simulink model "objselect"  (R2016a)
settings: Solver=VariableStepAuto  StartTime=0.0  StopTime=10.0  RelTol=1e-3
settings Model: Creator=NBGD  LastModifiedBy=NBGD

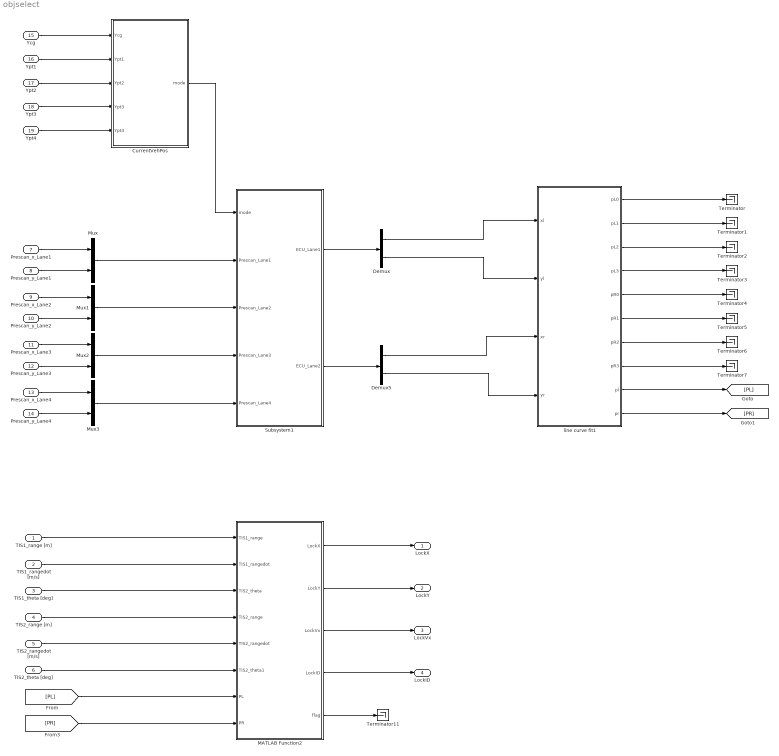
== system objselect ==
  TIS1_range [m] : Inport
  TIS1_rangedot [m/s] : Inport  Port=2
  TIS1_theta [deg] : Inport  Port=3
  TIS2_range [m] : Inport  Port=4
  TIS2_rangedot [m/s] : Inport  Port=5
  TIS2_theta [deg] : Inport  Port=6
  Prescan_x_Lane1 : Inport  Port=7
  Prescan_y_Lane1 : Inport  Port=8
  Prescan_x_Lane2 : Inport  Port=9
  Prescan_y_Lane2 : Inport  Port=10
  Prescan_x_Lane3 : Inport  Port=11
  Prescan_y_Lane3 : Inport  Port=12
  Prescan_x_Lane4 : Inport  Port=13
  Prescan_y_Lane4 : Inport  Port=14
  Ycg : Inport  Port=15
  Ypt1 : Inport  Port=16
  Ypt2 : Inport  Port=17
  Ypt3 : Inport  Port=18
  Ypt4 : Inport  Port=19
  CurrentVehPos : Subsystem
  Demux : Demux  Outputs=2
  Demux5 : Demux  Outputs=2
  MATLAB Function2 : MATLAB Function  TreatAsAtomicUnit=on
  Mux{,1..3} (4 alike) : Mux  Inputs=2
  Subsystem1 : Subsystem
  Terminator{,1..7,11} (9 alike) : Terminator
  line curve fit1 : MATLAB Function  TreatAsAtomicUnit=on
  LockX : Outport
  LockY : Outport  Port=2
  LockVx : Outport  Port=3
  LockID : Outport  Port=4
  wires:
  CurrentVehPos/1(mode) -> Subsystem1/1(mode)
  Demux/2 -> line curve fit1/2(yl)
  Demux5/2 -> line curve fit1/4(yr)
  Demux/1 -> line curve fit1/1(xl)
  Subsystem1/2(ECU_Lane2) -> Demux5/1
  line curve fit1/1(pL0) -> Terminator/1
  line curve fit1/2(pL1) -> Terminator1/1
  line curve fit1/3(pL2) -> Terminator2/1
  line curve fit1/4(pL3) -> Terminator3/1
  line curve fit1/5(pR0) -> Terminator4/1
  line curve fit1/6(pR1) -> Terminator5/1
  line curve fit1/7(pR2) -> Terminator6/1
  line curve fit1/8(pR3) -> Terminator7/1
  line curve fit1/9(pl) -> [PL]
  line curve fit1/10(pr) -> [PR]
  TIS1_range [m]/1 -> MATLAB Function2/1(TIS1_range)
  TIS1_rangedot [m/s]/1 -> MATLAB Function2/2(TIS1_rangedot)
  TIS1_theta [deg]/1 -> MATLAB Function2/3(TIS2_theta)
  TIS2_range [m]/1 -> MATLAB Function2/4(TIS2_range)
  TIS2_rangedot [m/s]/1 -> MATLAB Function2/5(TIS2_rangedot)
  TIS2_theta [deg]/1 -> MATLAB Function2/6(TIS2_theta1)
  MATLAB Function2/5(flag) -> Terminator11/1
  Prescan_x_Lane1/1 -> Mux/1
  Prescan_y_Lane1/1 -> Mux/2
  Mux/1 -> Subsystem1/2(Prescan_Lane1)
  Prescan_x_Lane2/1 -> Mux1/1
  Prescan_y_Lane2/1 -> Mux1/2
  Mux1/1 -> Subsystem1/3(Prescan_Lane2)
  Prescan_x_Lane3/1 -> Mux2/1
  Prescan_y_Lane3/1 -> Mux2/2
  Prescan_x_Lane4/1 -> Mux3/1
  Prescan_y_Lane4/1 -> Mux3/2
  Mux2/1 -> Subsystem1/4(Prescan_Lane3)
  Mux3/1 -> Subsystem1/5(Prescan_Lane4)
  Subsystem1/1(ECU_Lane1) -> Demux/1
  Demux5/1 -> line curve fit1/3(xr)
  [PL] -> MATLAB Function2/7(PL)
  [PR] -> MATLAB Function2/8(PR)
  MATLAB Function2/1(LockX) -> LockX/1
  MATLAB Function2/2(LockY) -> LockY/1
  MATLAB Function2/4(LockID) -> LockID/1
  MATLAB Function2/3(LockVx) -> LockVx/1
  Ycg/1 -> CurrentVehPos/1(Ycg)
  Ypt1/1 -> CurrentVehPos/2(Ypt1)
  Ypt2/1 -> CurrentVehPos/3(Ypt2)
  Ypt3/1 -> CurrentVehPos/4(Ypt3)
  Ypt4/1 -> CurrentVehPos/5(Ypt4)

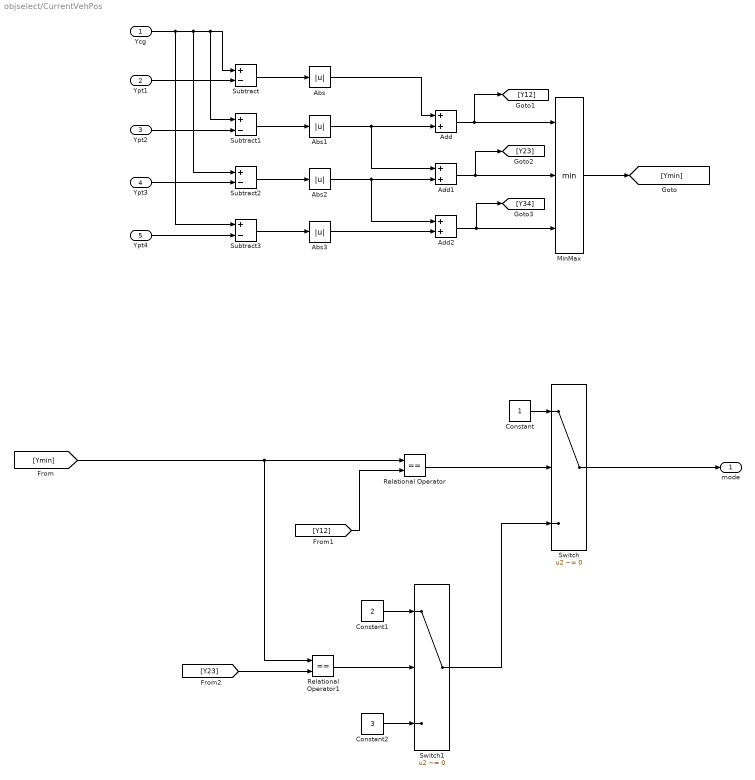
== system objselect/CurrentVehPos ==
  Ycg : Inport
  Ypt1 : Inport  Port=2
  Ypt2 : Inport  Port=3
  Ypt3 : Inport  Port=4
  Ypt4 : Inport  Port=5
  Abs{,1..3} (4 alike) : Abs
  Add : Sum
  Add1 : Sum
  Add2 : Sum
  Constant : Constant
  Constant1 : Constant  Value=2
  Constant2 : Constant  Value=3
  MinMax : MinMax  Inputs=3
  Relational Operator : RelationalOperator  Operator===  OutDataTypeStr=boolean
  Relational Operator1 : RelationalOperator  Operator===  OutDataTypeStr=boolean
  Subtract{,1..3} (4 alike) : Sum  Inputs=+-
  Switch : Switch  Criteria=u2 ~= 0
  Switch1 : Switch  Criteria=u2 ~= 0
  mode : Outport
  wires:
  Ycg/1 -> Subtract3/1, Subtract2/1, Subtract1/1, Subtract/1
  Abs/1 -> Add/1
  Ypt1/1 -> Subtract/2
  Subtract/1 -> Abs/1
  Ypt2/1 -> Subtract1/2
  Ypt3/1 -> Subtract2/2
  Ypt4/1 -> Subtract3/2
  Subtract2/1 -> Abs2/1
  Subtract3/1 -> Abs3/1
  Subtract1/1 -> Abs1/1
  Abs1/1 -> Add1/1, Add/2
  Abs2/1 -> Add2/1, Add1/2
  Abs3/1 -> Add2/2
  Add1/1 -> [Y23], MinMax/2
  Add/1 -> [Y12], MinMax/1
  Add2/1 -> [Y34], MinMax/3
  MinMax/1 -> [Ymin]
  Constant/1 -> Switch/1
  [Ymin] -> Relational Operator1/1, Relational Operator/1
  [Y12] -> Relational Operator/2
  Relational Operator/1 -> Switch/2
  Switch1/1 -> Switch/3
  Constant1/1 -> Switch1/1
  Relational Operator1/1 -> Switch1/2
  [Y23] -> Relational Operator1/2
  Constant2/1 -> Switch1/3
  Switch/1 -> mode/1

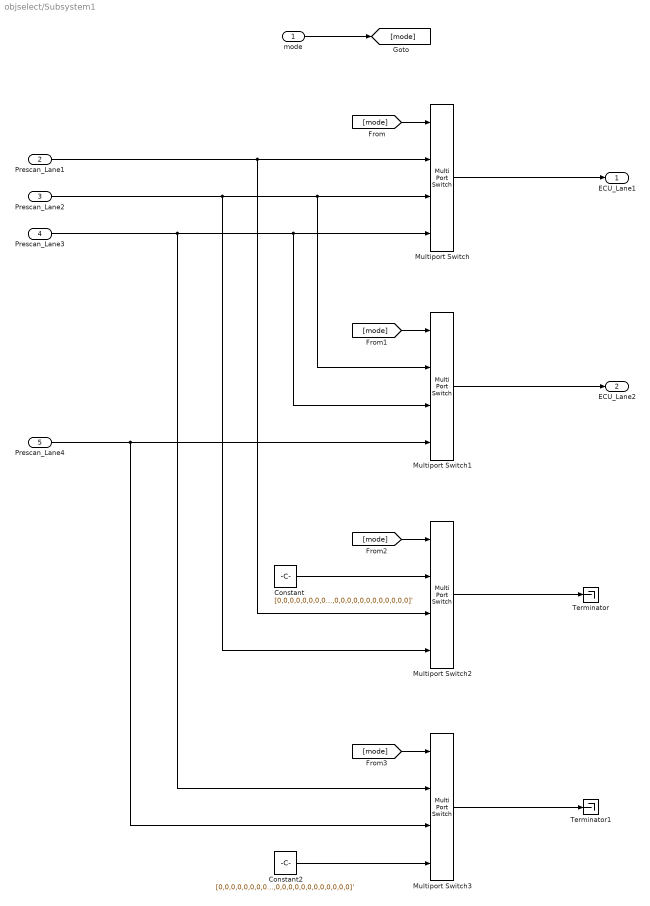
== system objselect/Subsystem1 ==
  mode : Inport
  Prescan_Lane1 : Inport  Port=2
  Prescan_Lane2 : Inport  Port=3
  Prescan_Lane3 : Inport  Port=4
  Prescan_Lane4 : Inport  Port=5
  Constant : Constant  Value=[0,0,0,0,0,0,0,0,0,0,0,0,0,0,0,0,0,0,0,0]'
  Constant2 : Constant  Value=[0,0,0,0,0,0,0,0,0,0,0,0,0,0,0,0,0,0,0,0]'
  Multiport Switch{,1..3} (4 alike) : MultiPortSwitch
  Terminator : Terminator
  Terminator1 : Terminator
  ECU_Lane1 : Outport
  ECU_Lane2 : Outport  Port=2
  wires:
  [mode] -> Multiport Switch/1
  Prescan_Lane1/1 -> Multiport Switch2/3, Multiport Switch/2
  Multiport Switch/1 -> ECU_Lane1/1
  [mode] -> Multiport Switch1/1
  Multiport Switch1/1 -> ECU_Lane2/1
  Prescan_Lane4/1 -> Multiport Switch3/3, Multiport Switch1/4
  mode/1 -> [mode]
  [mode] -> Multiport Switch2/1
  Constant/1 -> Multiport Switch2/2
  Multiport Switch2/1 -> Terminator/1
  Prescan_Lane2/1 -> Multiport Switch2/4, Multiport Switch1/2, Multiport Switch/3
  [mode] -> Multiport Switch3/1
  Prescan_Lane3/1 -> Multiport Switch3/2, Multiport Switch1/3, Multiport Switch/4
  Multiport Switch3/1 -> Terminator1/1
  Constant2/1 -> Multiport Switch3/4

== matlab function objselect/line curve fit1 ==
  data: xl input; pL0 output; yl input; xr input; pL1 output; yr input; pL2 output; pL3 output; pR0 output; pR1 output; pR2 output; pR3 output; pl output; pr output
function [pL0,pL1,pL2,pL3,pR0,pR1,pR2,pR3,pl,pr] = fcn(xl,yl,xr,yr)
%#eml
% pL3 = 0;
% pL2 = 0;
% pL1 = 0;
% pL0 = 0;
% pR3 = 0;
% pR2 = 0;
% pR1 = 0;
% pR0 = 0;

[pl,Sl] = polyfit(xl,yl,3);
pL3 = pl(1);
pL2 = pl(2);
pL1 = pl(3);
pL0 = pl(4);
[pr,Sr] = polyfit(xr,yr,3);
pR3 = pr(1);
pR2 = pr(2);
pR1 = pr(3);
pR0 = pr(4);

if isnan(pL3)
    pL3 = 0;
    pL2 = 0;
    pL1 = 0;
    pL0 = 0;  
end

if isnan(pR3)
    pR3 = 0;
    pR2 = 0;
    pR1 = 0;
    pR0 = 0;  
end

== matlab function objselect/MATLAB Function2 ==
  data: TIS1_range input; LockX output; TIS1_rangedot input; TIS2_theta input; TIS2_range input; TIS2_rangedot input; TIS2_theta1 input; PL input; PR input; LockY output; LockVx output; LockID output; flag output
function [LockX,LockY,LockVx,LockID,flag] = fcn(TIS1_range,TIS1_rangedot,TIS2_theta,TIS2_range,TIS2_rangedot,TIS2_theta1,PL,PR)
%#codegen

% if T==3.6
%     falg=1;
% end
TIS_range    = [TIS1_range,TIS2_range];
TIS_rangedot = [TIS1_rangedot,TIS2_rangedot];
TIS_theta    = [TIS1_theta,TIS2_theta]*pi()/180;
obj_x        = TIS_range .* cos(TIS_theta);
obj_y        = TIS_range .* sin(TIS_theta);
fitA_y       = polyval(PL,obj_x);
fitB_y       = polyval(PR,obj_x);
flag = 0;
%% make the points to several group

index1      = obj_x>0.01;                               %object in sensor range
index2      = obj_y<=fitA_y & obj_y>=fitB_y & index1;    %object in ego car lane 

if any(index2)~=0;                              %be sure has object in trace
    flag = 1;
    id_xmin           = find(obj_x==min(obj_x(index2)));            %the nearist object in detected
    id_xmin_intrace   = id_xmin(find(index2(id_xmin)==true));       %the nearist object in trace
    LockID            = min(id_xmin_intrace);                       %if more than 2 points get the low ID number
    LockX             = obj_x(LockID);
    LockY             = obj_y(LockID);
    LockVx            = TIS_rangedot(LockID);
else
    LockID            = 0;
    LockX             = 255;
    LockY             = 0;
    LockVx            = 0;
end
